simulink model "aoa_ekfmodel"  (R2019a)
settings: Solver=VariableStepAuto  StartTime=0.0  StopTime=7  RelTol=1e-3
libraries: simulink_extras x1
settings Model: Creator=phand  LastModifiedBy=phand

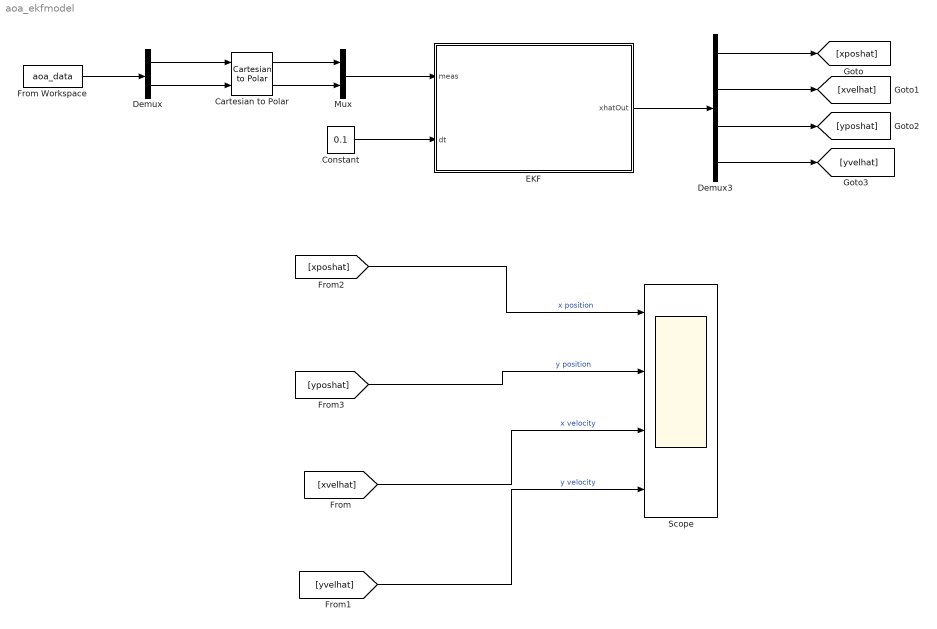
== system aoa_ekfmodel ==
  Cartesian to Polar : simulink_extras/Transformations/Cartesian to Polar
      settings: SourceProductName=Simulink
  Constant : Constant  Value=0.1
  Demux : Demux  Outputs=2
  Demux3 : Demux
  "EKF " : MATLAB Function  TreatAsAtomicUnit=on
  From Workspace : FromWorkspace  VariableName=aoa_data  SampleTime=0
  Mux : Mux  Inputs=2
  Scope : Scope  NumInputPorts=4
  wires:
  From Workspace/1 -> Demux/1
  Demux/2 -> Cartesian to Polar/2
  Demux/1 -> Cartesian to Polar/1
  Cartesian to Polar/2 -> Mux/2
  Cartesian to Polar/1 -> Mux/1
  Mux/1 -> "EKF "/1(meas)
  Constant/1 -> "EKF "/2(dt)
  Demux3/2 -> [xvelhat]
  Demux3/3 -> [yposhat]
  Demux3/1 -> [xposhat]
  "EKF "/1(xhatOut) -> Demux3/1
  Demux3/4 -> [yvelhat]
  [yposhat] -> Scope/2  "y position"
  [xposhat] -> Scope/1  "x position"
  [xvelhat] -> Scope/3  "x velocity"
  [yvelhat] -> Scope/4  "y velocity"

== matlab function aoa_ekfmodel/EKF  ==
  settings: updateMethod=DISCRETE
  data: meas input; xhatOut output; dt input
function xhatOut = EKF(meas, dt)
% This Embedded MATLAB Function implements an extended Kalman filter used
% for object tracking.
%
% The states of the process are given by
% x = [x_position; x_velocity; y_position; y_velocity];
%
% and the measurements are given by
% y = [range; bearing]
%
% where 
% range = sqrt(x_position^2 + y_position^2)
% bearing = atan2(y_position/x_position)

% Author: Phil Goddard (phil@goddardconsulting.ca)
% Date: Q2, 2011.

% Define storage for the variables that need to persist
% between time periods.
persistent P xhat Q R
if isempty(P)
    %[xvel, yvel] = acc_init(35);
    %[xpos, ypos] = aoa_init(35);
    %[xinit, yinit] = acc_init(35);
    %[xposinit, yposinit] = aoa_init(35);
    xpos = 3;
    %xvel = 3.5;
    ypos = 4.2;
    %yvel = 1.2;
    
    % First time through the code so do some initialization
    xhat = [0.1; 0.1; 0.1; 0.1];
    %xhat = [-900;80;950;20];
    P = zeros(4,4);
    Q =  diag([0.3 0.6 0.3 0.6]);
    R =  diag([0.25 0.25]);
end
% Calculate the Jacobians for the state and measurement equations
F = [1 dt 0 0;0 1 0 0;0 0 1 dt;0 0 0 1];
rangeHat = sqrt(xhat(1)^2+xhat(3)^2);
bearingHat = atan2(xhat(3),xhat(1));
yhat = [rangeHat; bearingHat]; 
H = [cos(bearingHat) 0 sin(bearingHat) 0;
    -sin(bearingHat)/rangeHat 0 cos(bearingHat)/rangeHat 0];

% Propogate the state and covariance matrices
xhat = F*xhat;
P = F*P*F' + Q;

% Calculate the Kalman gain
K = P*H'/(H*P*H' + R);

% Calculate the measurement residual
resid = meas - yhat;

% Update the state and covariance estimates
xhat = xhat + K*resid;
P = (eye(size(K,1))-K*H)*P;

% Post the results
xhatOut = xhat;
